simulink model "SystemBlock"  (R2022a)
settings: Solver=VariableStepAuto  StartTime=0.0  StopTime=10.0  RelTol=1e-3
undefined symbols (not defined in the file): I_xx, I_yy, I_zz, K1, K2, K3, K4, m
settings Model: SimulationMode=accelerator  Creator=Pascal  LastModifiedBy=wheel
settings SolverCC: AlgebraicLoopSolver=TrustRegion
settings DataIOCC: ReturnWorkspaceOutputs=off
settings DebuggingCC: UnconnectedInputMsg=warning  UnconnectedOutputMsg=warning  UnconnectedLineMsg=warning  SFMachineParentedDataDiag=warning  ArithmeticOperatorsInVariantConditions=warning
settings SFSimCC: CustomCodeUndefinedFunction=UseInterfaceOnly

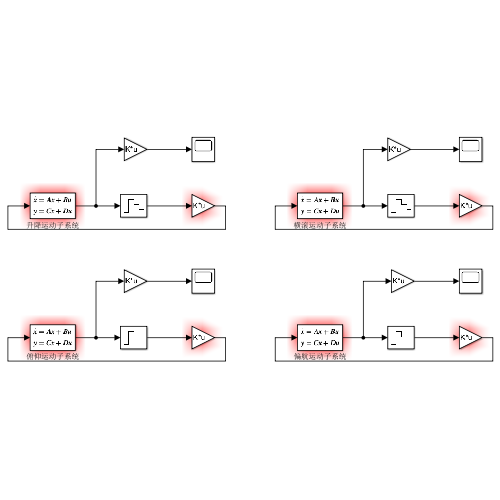
[thumbnail: Simulink's stored preview of the top-level diagram]
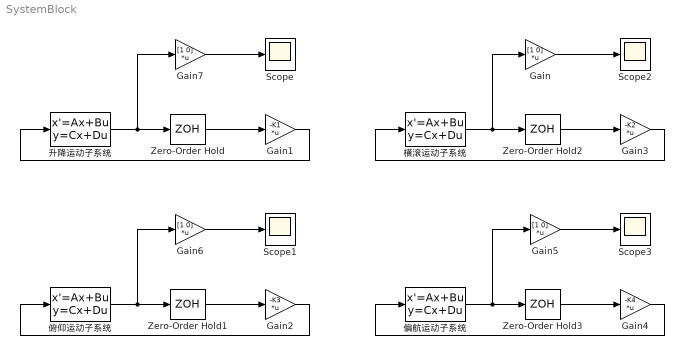
== system SystemBlock ==
  Gain{,5..7} (4 alike) : Gain  Gain=[1 0]  Multiplication=Matrix(K*u)
  Gain1 : Gain  Gain=-K1  Multiplication=Matrix(K*u)
  Gain2 : Gain  Gain=-K3  Multiplication=Matrix(K*u)
  Gain3 : Gain  Gain=-K2  Multiplication=Matrix(K*u)
  Gain4 : Gain  Gain=-K4  Multiplication=Matrix(K*u)
  Scope{,1..3} (4 alike) : Scope
  Zero-Order Hold{,1..3} (4 alike) : ZeroOrderHold  SampleTime=0.005
  俯仰运动子系统 : StateSpace  A=[0 1; 0 0]  B=[0; 1/I_yy]  C=eye(2)  D=zeros(2,1)  InitialCondition=[0.0873; 0]
  偏航运动子系统 : StateSpace  A=[0 1; 0 0]  B=[0; 1/I_zz]  C=eye(2)  D=zeros(2,1)  InitialCondition=[0.0873; 0]
  升降运动子系统 : StateSpace  A=[0 1; 0 0]  B=[0; 1/m]  C=eye(2)  D=zeros(2,1)  InitialCondition=[-1; 0]
  横滚运动子系统 : StateSpace  A=[0 1; 0 0]  B=[0; 1/I_xx]  C=eye(2)  D=zeros(2,1)  InitialCondition=[0.0873; 0]
  wires:
  升降运动子系统/1 -> Gain7/1, Zero-Order Hold/1
  Zero-Order Hold/1 -> Gain1/1
  Gain1/1 -> 升降运动子系统/1
  俯仰运动子系统/1 -> Gain6/1, Zero-Order Hold1/1
  Zero-Order Hold1/1 -> Gain2/1
  Gain2/1 -> 俯仰运动子系统/1
  横滚运动子系统/1 -> Gain/1, Zero-Order Hold2/1
  Zero-Order Hold2/1 -> Gain3/1
  Gain3/1 -> 横滚运动子系统/1
  Zero-Order Hold3/1 -> Gain4/1
  Gain4/1 -> 偏航运动子系统/1
  偏航运动子系统/1 -> Gain5/1, Zero-Order Hold3/1
  Gain/1 -> Scope2/1
  Gain5/1 -> Scope3/1
  Gain6/1 -> Scope1/1
  Gain7/1 -> Scope/1
